simulink model "ExampleSystem"  (R2015b)
settings: Solver=VariableStepAuto  StartTime=0.0  StopTime=10.0  RelTol=1e-3
settings Model: Creator=u265735  LastModifiedBy=u265735
settings ConfigComp: CovModelRefEnable=Off

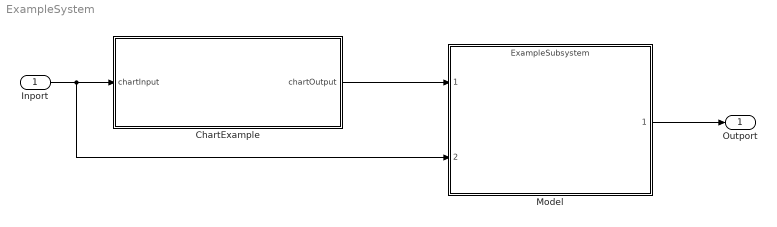
== system ExampleSystem ==
  Inport : Inport
  ChartExample : Stateflow chart  TreatAsAtomicUnit=on
  Model : ModelReference  ModelNameDialog=ExampleSubsystem.slx  SimulationMode=Normal  ModelReferenceVersion=1.1  CopyOfModelName=ExampleSubsystem.slx
  Outport : Outport
  wires:
  Inport/1 -> Model/2, ChartExample/1(chartInput)
  ChartExample/1(chartOutput) -> Model/1
  Model/1 -> Outport/1

== stateflow chart ExampleSystem/ChartExample ==
  state Hello
    state World
    (default) -> World
  (default) -> Hello
  data: chartInput input; chartOutput output
